simulink model "sampleModel275"  (R2021b)
settings: Solver=VariableStepAuto  StartTime=0.0  StopTime=10.0  RelTol=1e-3
undefined symbols (not defined in the file or in its folder): DiscIntNeverNeededParam, Newton, Raphson
libraries: simulink x15, slpidlib x3
settings Model: Creator=user  LastModifiedBy=user

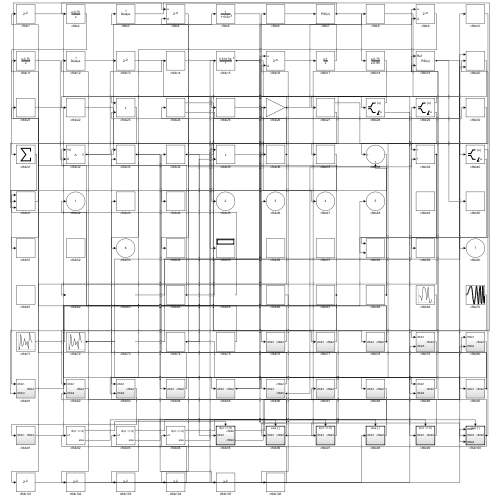
[thumbnail: Simulink's stored preview of the top-level diagram]
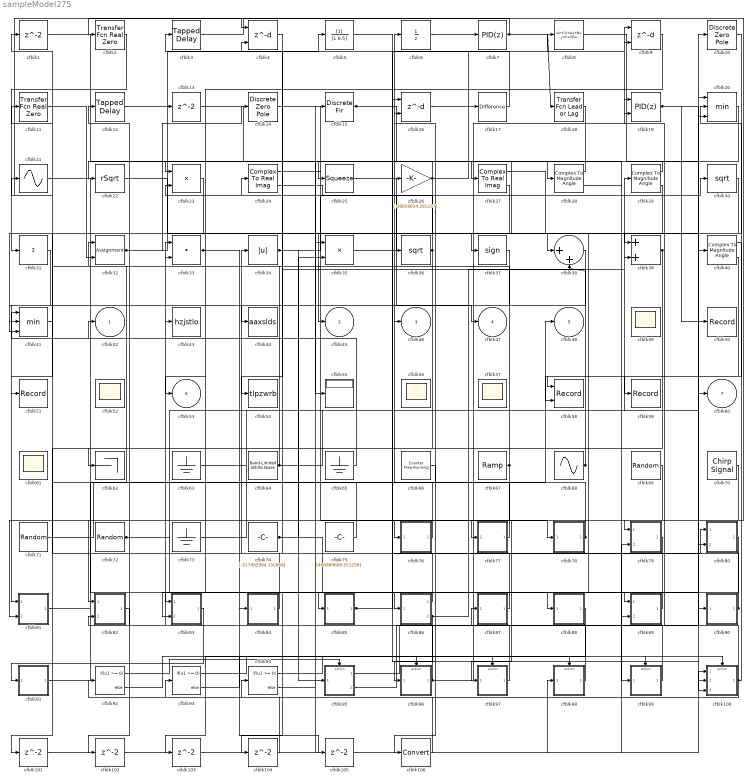
== system sampleModel275 ==
  cfblk{1,13,101..105} (7 alike) : Delay  SampleTime=1
  cfblk10 : DiscreteZeroPole  Poles=[0 0.5]  Gain=1
  cfblk100 : Subsystem  TreatAsAtomicUnit=on
  cfblk106 : DataTypeConversion
  cfblk11 : simulink/Discrete/Transfer Fcn Real Zero  ZeroZ=0.75  ICPrevInput=0.0  DoSatur=off
      settings: SourceProductBaseCode=SL
  cfblk12 : simulink/Discrete/Tapped Delay  vinit=0.0  samptime=-1  NumDelays=1  DelayOrder=Oldest  includeCurrent=off
  cfblk14 : DiscreteZeroPole  Poles=[0 0.5]  Gain=1
  cfblk15 : DiscreteFir  SampleTime=1
  cfblk16 : Delay  DelayLengthSource=Input port  SampleTime=1
      settings: InputPortMap=u0,p1
  cfblk17 : simulink/Discrete/Difference  ICPrevInput=0.0  OutMin=[]  OutMax=[]  OutDataTypeStr=Inherit: Inherit via back propagation  OutDataType=fixdt(1, 16)  OutScaling=2^-10  DoSatur=off
  cfblk18 : simulink/Discrete/Transfer Fcn Lead or Lag  PoleZ=0.95  ZeroZ=0.75  ICPrevOutput=0.0  ICPrevInput=0.0  DoSatur=off
      settings: SourceProductBaseCode=SL
  cfblk19 : slpidlib/PID Controller (2DOF)  Controller=PID  Form=Parallel  TimeDomain=Discrete-time  UseExternalTs=off  SampleTime=1  IntegratorMethod=Forward Euler  FilterMethod=Forward Euler  ControllerParametersSource=internal  P=1  I=1  D=0  UseFilter=on  N=100  b=1  c=1  TunerSelectOption=Transfer Function Based (PID Tuner App)  InitialConditionSource=internal  InitialConditionForIntegrator=0  InitialConditionForFilter=0  DifferentiatorICPrevScaledInput=0  ExternalReset=none  TrackingMode=off  Kt=1  LimitOutput=off  SatLimitsSource=internal  UpperSaturationLimit=inf  LowerSaturationLimit=-inf  LinearizeAsGain=off  AntiWindupMode=none  Kb=1  POutMin=[]  POutMax=[]  IOutMin=[]  IOutMax=[]  DOutMin=[]  DOutMax=[]  NOutMin=[]  NOutMax=[]  bOutMin=[]  bOutMax=[]  cOutMin=[]  cOutMax=[]  SumOutMin=[]  SumOutMax=[]  SaturationOutMin=[]  SaturationOutMax=[]  PParamMin=[]  PParamMax=[]  IParamMin=[]  IParamMax=[]  DParamMin=[]  DParamMax=[]  NParamMin=[]  NParamMax=[]  bParamMin=[]  bParamMax=[]  cParamMin=[]  cParamMax=[]  KbParamMin=[]  KbParamMax=[]  KtParamMin=[]  KtParamMax=[]  KbOutMin=[]  KbOutMax=[]  KtOutMin=[]  KtOutMax=[]  IntegratorOutMin=[]  IntegratorOutMax=[]  FilterOutMin=[]  FilterOutMax=[]  SumI1OutMin=[]  SumI1OutMax=[]  SumI2OutMin=[]  SumI2OutMax=[]  SumI3OutMin=[]  SumI3OutMax=[]  SumI4OutMin=[]  SumI4OutMax=[]  SumDOutMin=[]  SumDOutMax=[]  Sum1OutMin=[]  Sum1OutMax=[]  Sum2OutMin=[]  Sum2OutMax=[]  Sum3OutMin=[]  Sum3OutMax=[]  DifferentiatorOutMin=[]  DifferentiatorOutMax=[]  FilterDiffOutCoefMin=[]  FilterDiffOutCoefMax=[]  ReciprocalOutMin=[]  ReciprocalOutMax=[]  SumDenOutMin=[]  SumDenOutMax=[]  SumNumOutMin=[]  SumNumOutMax=[]  DivideOutMin=[]  DivideOutMax=[]  UdiffTsProdOutMin=[]  UdiffTsProdOutMax=[]  NTsProdOutMin=[]  NTsProdOutMax=[]  UintegralTsProdOutMin=[]  UintegralTsProdOutMax=[]  UngainTsProdOutMin=[]  UngainTsProdOutMax=[]  IntegratorContinuousStateAttributes=''  IntegratorStateMustResolveToSignalObject=off  IntegratorRTWStateStorageClass=Auto  FilterContinuousStateAttributes=''  FilterStateMustResolveToSignalObject=off  FilterRTWStateStorageClass=Auto  ParallelPVariant=InternalParameters  IdealPVariant=Disabled  IVariant=InternalParameters  DVariant=InternalParameters  bVariant=InternalParameters  cVariant=InternalParameters  IntegratorVariant=Discrete  SatVariant=Disabled  AWVariant=Passthrough  PCopyVariant=Disabled  TRVariant=Disabled  FdbkBlocksVariant=Forward  IdealPFdbkVariant=Disabled  SatFdbkVariant=Disabled  DerivativeFilterVariant=ForwardEulerFilter  NVariant=InternalParameters  NCopyVariant=Disabled  FilterICVariant=InternalICsFilter  IntegratorICVariant=InternalICs  ExternalResetVariant=Disabled  TRSumVariant=Passthrough  SumFdbkVariant=Disabled  SumVariant=Sum_PID  TsampFilterVariant=InternalTs  TsampNgainVariant=Passthrough  TsampIntegralVariant=Passthrough  ExternalSaturationOutDataTypeStr=Inherit: Same as second input
      settings: SourceProductBaseCode=SL
  cfblk2 : simulink/Discrete/Transfer Fcn Real Zero  ZeroZ=0.75  ICPrevInput=0.0  DoSatur=off
      settings: SourceProductBaseCode=SL
  cfblk20 : MinMax  Inputs=3
  cfblk21 : Sin  TimeSource=Use external signal  SampleTime=0
  cfblk22 : Sqrt  Operator=rSqrt  AlgorithmType=Newton-Raphson  SaturateOnIntegerOverflow=on
  cfblk23 : Product
  cfblk24 : ComplexToRealImag
  cfblk25 : Squeeze
  cfblk26 : Gain  Gain=[-28658814.291237]
  cfblk27 : ComplexToRealImag
  cfblk28 : ComplexToMagnitudeAngle
  cfblk29 : ComplexToMagnitudeAngle
  cfblk3 : simulink/Discrete/Tapped Delay  vinit=0.0  samptime=-1  NumDelays=1  DelayOrder=Oldest  includeCurrent=off
  cfblk30 : Sqrt  SaturateOnIntegerOverflow=on
  cfblk31 : Sum  Inputs=+
  cfblk32 : Assignment  DiagnosticForDimensions=Warning  IndexOptions=Index vector (dialog)  Indices=1  OutputSizes=1
  cfblk33 : DotProduct  InputSameDT=on  OutDataTypeStr=Inherit: Inherit via internal rule
  cfblk34 : Abs
  cfblk35 : Product  Inputs=**
  cfblk36 : Sqrt  SaturateOnIntegerOverflow=on
  cfblk37 : Signum
  cfblk38 : Sum  Inputs=|++
  cfblk39 : Sum
  cfblk4 : Delay  DelayLengthSource=Input port  SampleTime=1
      settings: InputPortMap=u0,p1
  cfblk40 : ComplexToMagnitudeAngle
  cfblk41 : MinMax  Inputs=3
  cfblk43 : ToWorkspace  VariableName=hzjstlo  SaveFormat=Timeseries  SampleTime=-1
  cfblk44 : ToWorkspace  VariableName=aaxslds  SaveFormat=Timeseries  SampleTime=-1
  cfblk{49,52,56..57,61} (5 alike) : Scope
      settings: Floating=on
  cfblk5 : DiscreteFilter  SampleTime=1
  cfblk50 : Record  FileSettingsInternal="{\"entries\":[{\"content\":{\"excelSettings\":{\"content\":{},\"type\":\"Streamout.ExcelSettings\"}},\"type\":\"Streamout.FileSettingStorage\",\"uuid\":\"b6eb8a9c-eb1a-4261-9b81-98630c569aa1\"}],\"packageUris\":[\"http://schema.mathworks.com/mf0/streamout_blocks/R2020a\"],\"version\":\"1.0\"}"  SignalsInternal="{\"entries\":[{\"content\":{\"signals\":[{\"content\":{\"blockPath\":[\"sampleModel275/cfblk50\"],\"channel\":[],\"dimensions\":[1],\"domain\":\"sampleModel275/cfblk50\",\"lineColor\":\"#fe330a\",\"plots\":[1],\"port\":1,\"sid\":[\"\"],\"signalID\":11495,\"signalName\":\"cfblk19\"},\"type\":\"RecordBlkView.Signal\",\"uuid\":\"71f57f67-cb61-4adf-8332-56198fc03cd2\"}]},\"type\":\"RecordBlkView.InputSignals\",\"uuid\":\"8c8ca269-4e9b-46e2-88c4-c1c2e234a8b1\"}],\"packageUris\":[\"http://schema.mathworks.com/mf0/streamout_blocks/R2020a\"],\"version\":\"1.0\"}"  VisualizationBindings="{\"sparklinesplugin\":{\"info\":[{\"bindingParametersList\":[],\"subplotID\":1}]}}"
  cfblk51 : Record  FileSettingsInternal="{\"entries\":[{\"content\":{\"excelSettings\":{\"content\":{},\"type\":\"Streamout.ExcelSettings\"}},\"type\":\"Streamout.FileSettingStorage\",\"uuid\":\"b407e88e-82d7-4c58-97ca-e59b3c794d53\"}],\"packageUris\":[\"http://schema.mathworks.com/mf0/streamout_blocks/R2020a\"],\"version\":\"1.0\"}"  SignalsInternal="{\"entries\":[{\"content\":{\"signals\":[{\"content\":{\"blockPath\":[\"sampleModel275/cfblk51\"],\"channel\":[],\"dimensions\":[1],\"domain\":\"sampleModel275/cfblk51\",\"lineColor\":\"#22b573\",\"plots\":[1],\"port\":1,\"sid\":[\"\"],\"signalID\":11499,\"signalName\":\"cfblk23\"},\"type\":\"RecordBlkView.Signal\",\"uuid\":\"ec15170a-8382-47db-b36d-1ce41cc8f111\"}]},\"type\":\"RecordBlkView.InputSignals\",\"uuid\":\"f86542a5-57eb-4307-8b55-610ba7e4df7d\"}],\"packageUris\":[\"http://schema.mathworks.com/mf0/streamout_blocks/R2020a\"],\"version\":\"1.0\"}"  VisualizationBindings="{\"sparklinesplugin\":{\"info\":[{\"bindingParametersList\":[],\"subplotID\":1}]}}"
  cfblk54 : ToWorkspace  VariableName=tlpzwrb  SaveFormat=Timeseries  SampleTime=-1
  cfblk55 : Display
  cfblk58 : Record  FileSettingsInternal="{\"entries\":[{\"content\":{\"excelSettings\":{\"content\":{},\"type\":\"Streamout.ExcelSettings\"}},\"type\":\"Streamout.FileSettingStorage\",\"uuid\":\"6438ada9-0782-4b46-9d9c-291e916b62cd\"}],\"packageUris\":[\"http://schema.mathworks.com/mf0/streamout_blocks/R2020a\"],\"version\":\"1.0\"}"  Layout=[1 1]  SignalsInternal="{\"entries\":[{\"content\":{\"signals\":[{\"content\":{\"blockPath\":[\"sampleModel275/cfblk58\"],\"channel\":[],\"dimensions\":[1],\"domain\":\"sampleModel275/cfblk58\",\"lineColor\":\"#a2142f\",\"plots\":[1],\"port\":1,\"sid\":[\"\"],\"signalID\":11503,\"signalName\":\"cfblk40:1\"},\"type\":\"RecordBlkView.Signal\",\"uuid\":\"d4910d3c-664b-4734-92f5-20726efe3d51\"},{\"content\":{\"blockPath\":[\"sampleModel275/cfblk58\"],\"channel\":[],\"dimensions\":[1],\"domain\":\"sampleModel275/cfblk58\",\"lineColor\":\"#139fff\",\"plots\":[1],\"port\":2,\"sid\":[\"\"],\"signalID\":11507,\"signalName\":\"cfblk39\"},\"type\":\"RecordBlkView.Signal\",\"uuid\":\"d5fbbb1f-5277-447b-a33f-a90c886777ef\"}]},\"type\":\"RecordBlkView.InputSignals\",\"uuid\":\"5aa0f4f9-8f77-40f4-b90e-7cbebfc535ff\"}],\"packageUris\":[\"http://schema.mathworks.com/mf0/streamout_blocks/R2020a\"],\"version\":\"1.0\"}"  VisualizationBindings="{\"xyplotplugin\":{\"info\":[{\"series\":[{\"bindingParametersList\":[{\"parameter\":\"X-Axis\",\"signalID\":11503,\"signalName\":\"cfblk40:1\"},{\"parameter\":\"Y-Axis\",\"signalID\":11507,\"signalName\":\"cfblk39\"}],\"seriesID\":64902}],\"subplotID\":1}]}}"  CompatibilityTag=XY
  cfblk59 : Record  FileSettingsInternal="{\"entries\":[{\"content\":{\"excelSettings\":{\"content\":{},\"type\":\"Streamout.ExcelSettings\"}},\"type\":\"Streamout.FileSettingStorage\",\"uuid\":\"0cc106a6-c31f-4d23-977d-6d8b87a6092b\"}],\"packageUris\":[\"http://schema.mathworks.com/mf0/streamout_blocks/R2020a\"],\"version\":\"1.0\"}"  SignalsInternal="{\"entries\":[{\"content\":{\"signals\":[{\"content\":{\"blockPath\":[\"sampleModel275/cfblk59\"],\"channel\":[],\"dimensions\":[1],\"domain\":\"sampleModel275/cfblk59\",\"lineColor\":\"#edb120\",\"plots\":[1],\"port\":1,\"sid\":[\"\"],\"signalID\":11511,\"signalName\":\"cfblk40:2\"},\"type\":\"RecordBlkView.Signal\",\"uuid\":\"fdcc7cc7-3bfd-4a9a-aeaa-3b1704c8eba9\"}]},\"type\":\"RecordBlkView.InputSignals\",\"uuid\":\"85a8b503-552f-41f1-b276-6a567ca8898e\"}],\"packageUris\":[\"http://schema.mathworks.com/mf0/streamout_blocks/R2020a\"],\"version\":\"1.0\"}"  VisualizationBindings="{\"sparklinesplugin\":{\"info\":[{\"bindingParametersList\":[],\"subplotID\":1}]}}"
  cfblk6 : UnitDelay  HasFrameUpgradeWarning=on
  cfblk62 : Terminator
  cfblk63 : Ground
  cfblk64 : simulink/Sources/Band-Limited White Noise  Cov=[1822602826.106394]  Ts=0.1  seed=[609401567.000000]
  cfblk65 : Ground
  cfblk66 : simulink/Sources/Counter Free-Running  NumBits=[2.000000]  tsamp=-1
  cfblk67 : simulink/Sources/Ramp  slope=[-6244.976226]  start=[33.233688]  InitialOutput=[-507448.704039]
  cfblk68 : Sin  Amplitude=[-991310042.468495]  Bias=[911881758.142677]  SampleTime=0
  cfblk69 : RandomNumber  Mean=[-38034.714186]  Variance=[20282.555075]  Seed=[711987577.000000]  SampleTime=0.1
  cfblk7 : slpidlib/PID Controller  Controller=PID  Form=Parallel  TimeDomain=Discrete-time  UseExternalTs=off  SampleTime=1  IntegratorMethod=Forward Euler  FilterMethod=Forward Euler  ControllerParametersSource=internal  P=1  I=1  D=0  UseFilter=on  N=100  TunerSelectOption=Transfer Function Based (PID Tuner App)  InitialConditionSource=internal  InitialConditionForIntegrator=0  InitialConditionForFilter=0  DifferentiatorICPrevScaledInput=0  ExternalReset=none  TrackingMode=off  Kt=1  LimitOutput=off  SatLimitsSource=internal  UpperSaturationLimit=inf  LowerSaturationLimit=-inf  LinearizeAsGain=off  AntiWindupMode=none  Kb=1  POutMin=[]  POutMax=[]  IOutMin=[]  IOutMax=[]  DOutMin=[]  DOutMax=[]  NOutMin=[]  NOutMax=[]  SumOutMin=[]  SumOutMax=[]  SaturationOutMin=[]  SaturationOutMax=[]  PParamMin=[]  PParamMax=[]  IParamMin=[]  IParamMax=[]  DParamMin=[]  DParamMax=[]  NParamMin=[]  NParamMax=[]  KbParamMin=[]  KbParamMax=[]  KtParamMin=[]  KtParamMax=[]  KbOutMin=[]  KbOutMax=[]  KtOutMin=[]  KtOutMax=[]  IntegratorOutMin=[]  IntegratorOutMax=[]  FilterOutMin=[]  FilterOutMax=[]  SumI1OutMin=[]  SumI1OutMax=[]  SumI2OutMin=[]  SumI2OutMax=[]  SumI3OutMin=[]  SumI3OutMax=[]  SumI4OutMin=[]  SumI4OutMax=[]  SumDOutMin=[]  SumDOutMax=[]  DifferentiatorOutMin=[]  DifferentiatorOutMax=[]  FilterDiffOutCoefMin=[]  FilterDiffOutCoefMax=[]  ReciprocalOutMin=[]  ReciprocalOutMax=[]  SumDenOutMin=[]  SumDenOutMax=[]  SumNumOutMin=[]  SumNumOutMax=[]  DivideOutMin=[]  DivideOutMax=[]  UdiffTsProdOutMin=[]  UdiffTsProdOutMax=[]  NTsProdOutMin=[]  NTsProdOutMax=[]  UintegralTsProdOutMin=[]  UintegralTsProdOutMax=[]  UngainTsProdOutMin=[]  UngainTsProdOutMax=[]  IntegratorContinuousStateAttributes=''  IntegratorStateMustResolveToSignalObject=off  IntegratorRTWStateStorageClass=Auto  FilterContinuousStateAttributes=''  FilterStateMustResolveToSignalObject=off  FilterRTWStateStorageClass=Auto  ParallelPVariant=InternalParameters  IdealPVariant=Disabled  IVariant=InternalParameters  DVariant=InternalParameters  IntegratorVariant=Discrete  SatVariant=Disabled  AWVariant=Passthrough  PCopyVariant=Disabled  TRVariant=Disabled  FdbkBlocksVariant=Forward  IdealPFdbkVariant=Disabled  SatFdbkVariant=Disabled  DerivativeFilterVariant=ForwardEulerFilter  NVariant=InternalParameters  NCopyVariant=Disabled  FilterICVariant=InternalICsFilter  IntegratorICVariant=InternalICs  ExternalResetVariant=Disabled  TRSumVariant=Passthrough  SumFdbkVariant=Disabled  SumVariant=Sum_PID  TsampFilterVariant=InternalTs  TsampNgainVariant=Passthrough  TsampIntegralVariant=Passthrough  ExternalSaturationOutDataTypeStr=Inherit: Same as second input
  cfblk70 : simulink/Sources/Chirp Signal  f1=[-497496428.255799]  T=[-926255871.400772]  f2=[-805731715.239342]
  cfblk71 : UniformRandomNumber  Minimum=[-1039848184.369478]  Maximum=[7342485115.905728]  Seed=[43463213.000000]  SampleTime=0.1
  cfblk72 : UniformRandomNumber  Minimum=[-2028484056.447849]  Maximum=[4927057979.813775]  Seed=[54197265.000000]  SampleTime=0.1
  cfblk73 : Ground
  cfblk74 : Constant  Value=[-527492994.150068]  SampleTime=1
  cfblk75 : Constant  Value=[406889608.551256]  SampleTime=1
  cfblk76 : Subsystem
  cfblk77 : Subsystem
  cfblk78 : Subsystem
  cfblk79 : Subsystem
  cfblk8 : DiscreteStateSpace
  cfblk80 : Subsystem
  cfblk81 : Subsystem
  cfblk82 : Subsystem
  cfblk83 : Subsystem
  cfblk84 : Subsystem
  cfblk85 : Subsystem
  cfblk86 : Subsystem
  cfblk87 : Subsystem
  cfblk88 : Subsystem
  cfblk89 : Subsystem
  cfblk9 : Delay  DelayLengthSource=Input port  SampleTime=1
      settings: InputPortMap=u0,p1
  cfblk90 : Subsystem
  cfblk91 : Subsystem
  cfblk92 : If  IfExpression=u1 >= 0  SampleTime=1
  cfblk93 : If  IfExpression=u1 >= 0  SampleTime=1
  cfblk94 : If  IfExpression=u1 >= 0  SampleTime=1
  cfblk95 : Subsystem  TreatAsAtomicUnit=on
  cfblk96 : Subsystem  TreatAsAtomicUnit=on
  cfblk97 : Subsystem  TreatAsAtomicUnit=on
  cfblk98 : Subsystem  TreatAsAtomicUnit=on
  cfblk99 : Subsystem  TreatAsAtomicUnit=on
  cfblk42 : Outport
  cfblk45 : Outport  Port=2
  cfblk46 : Outport  Port=3
  cfblk47 : Outport  Port=4
  cfblk48 : Outport  Port=5
  cfblk53 : Outport  Port=6
  cfblk60 : Outport  Port=7
  wires:
  cfblk17/1 -> cfblk3/1
  cfblk40/1 -> cfblk58/1
  cfblk21/1 -> cfblk85/1(cfblk1)
  cfblk96/1(cfblk2) -> cfblk9/1, cfblk82/2(cfblk4)
  cfblk71/1 -> cfblk48/1
  cfblk89/1(cfblk2) -> cfblk86/1(cfblk1)
  cfblk34/1 -> cfblk30/1, cfblk95/1(cfblk1)
  cfblk84/1(cfblk2) -> cfblk34/1
  cfblk3/1 -> cfblk79/1(cfblk1)
  cfblk24/1 -> cfblk76/1(cfblk1)
  cfblk10/1 -> cfblk38/1
  cfblk18/1 -> cfblk27/1
  cfblk14/1 -> cfblk77/1(cfblk1)
  cfblk32/1 -> cfblk5/1, cfblk14/1
  cfblk19/1 -> cfblk40/1, cfblk50/1
  cfblk73/1 -> cfblk6/1
  cfblk63/1 -> cfblk29/1
  cfblk20/1 -> cfblk37/1
  cfblk25/1 -> cfblk47/1
  cfblk24/2 -> cfblk26/1
  cfblk31/1 -> cfblk81/1(cfblk1)
  cfblk4/1 -> cfblk54/1
  cfblk97/1(cfblk2) -> cfblk33/1
  cfblk36/1 -> cfblk91/1(cfblk1), cfblk23/2
  cfblk37/1 -> cfblk44/1
  cfblk30/1 -> cfblk88/1(cfblk1)
  cfblk41/1 -> cfblk4/1
  cfblk90/1(cfblk2) -> cfblk4/2, cfblk19/2
  cfblk9/1 -> cfblk83/1(cfblk1)
  cfblk2/1 -> cfblk31/1
  cfblk65/1 -> cfblk41/1
  cfblk1/1 -> cfblk28/1
  cfblk39/1 -> cfblk62/1, cfblk58/2
  cfblk28/1 -> cfblk22/1
  cfblk33/1 -> cfblk84/1(cfblk1), cfblk105/1
  cfblk76/1(cfblk2) -> cfblk32/1
  cfblk26/1 -> cfblk45/1, cfblk25/1, cfblk9/2
  cfblk98/1(cfblk2) -> cfblk87/1(cfblk1)
  cfblk8/1 -> cfblk60/1
  cfblk67/1 -> cfblk33/2, cfblk82/1(cfblk1)
  cfblk70/1 -> cfblk81/2(cfblk3)
  cfblk87/1(cfblk2) -> cfblk1/1
  cfblk5/1 -> cfblk78/1(cfblk1)
  cfblk69/1 -> cfblk97/1(cfblk1)
  cfblk35/1 -> cfblk10/1
  cfblk22/1 -> cfblk90/1(cfblk1)
  cfblk85/1(cfblk2) -> cfblk80/1(cfblk1), cfblk8/1
  cfblk11/1 -> cfblk32/2
  cfblk23/1 -> cfblk51/1
  cfblk95/1(cfblk2) -> cfblk80/2(cfblk4)
  cfblk99/1(cfblk2) -> cfblk12/1
  cfblk74/1 -> cfblk89/1(cfblk1), cfblk35/2
  cfblk95/2(cfblk4) -> cfblk20/1
  cfblk77/1(cfblk2) -> cfblk46/1
  cfblk40/2 -> cfblk59/1
  cfblk64/1 -> cfblk16/1, cfblk21/1
  cfblk28/2 -> cfblk99/1(cfblk1)
  cfblk38/1 -> cfblk41/2
  cfblk78/1(cfblk2) -> cfblk42/1, cfblk16/2
  cfblk68/1 -> cfblk24/1, cfblk38/2
  cfblk72/1 -> cfblk100/2(cfblk3), cfblk20/3
  cfblk13/1 -> cfblk55/1
  cfblk15/1 -> cfblk89/2(cfblk4), cfblk100/3(cfblk4)
  cfblk6/1 -> cfblk7/1
  cfblk81/1(cfblk2) -> cfblk36/1
  cfblk12/1 -> cfblk13/1
  cfblk91/1(cfblk2) -> cfblk35/1
  cfblk29/1 -> cfblk23/1
  cfblk75/1 -> cfblk11/1
  cfblk27/1 -> cfblk39/1
  cfblk16/1 -> cfblk17/1
  cfblk27/2 -> cfblk41/3
  cfblk79/1(cfblk2) -> cfblk83/2(cfblk4)
  cfblk86/1(cfblk2) -> cfblk43/1
  cfblk29/2 -> cfblk53/1
  cfblk100/1(cfblk2) -> cfblk93/1, cfblk19/1, cfblk20/2
  cfblk86/2(cfblk5) -> cfblk96/1(cfblk1), cfblk39/2
  cfblk7/1 -> cfblk18/1, cfblk2/1
  cfblk92/1 -> cfblk95/Action
  cfblk92/2 -> cfblk96/Action
  cfblk93/1 -> cfblk97/Action
  cfblk93/2 -> cfblk98/Action
  cfblk94/1 -> cfblk99/Action
  cfblk94/2 -> cfblk100/Action
  cfblk83/1(cfblk2) -> cfblk101/1
  cfblk101/1 -> cfblk79/2(cfblk5)
  cfblk82/1(cfblk2) -> cfblk102/1
  cfblk102/1 -> cfblk15/1
  cfblk88/1(cfblk2) -> cfblk103/1
  cfblk103/1 -> cfblk100/1(cfblk1)
  cfblk80/1(cfblk2) -> cfblk104/1
  cfblk104/1 -> cfblk92/1
  cfblk105/1 -> cfblk98/1(cfblk1)
  cfblk66/1 -> cfblk106/1
  cfblk106/1 -> cfblk94/1

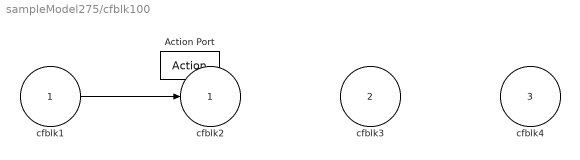
== system sampleModel275/cfblk100 ==
  cfblk1 : Inport
  cfblk3 : Inport  Port=2
  cfblk4 : Inport  Port=3
  Action Port : ActionPort  ActionPortLabel=else
  cfblk2 : Outport
  wires:
  cfblk1/1 -> cfblk2/1

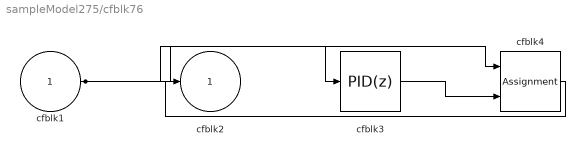
== system sampleModel275/cfblk76 ==
  cfblk1 : Inport
  cfblk3 : slpidlib/PID Controller  Controller=PID  Form=Parallel  TimeDomain=Discrete-time  UseExternalTs=off  SampleTime=1  IntegratorMethod=Forward Euler  FilterMethod=Forward Euler  ControllerParametersSource=internal  P=1  I=1  D=0  UseFilter=on  N=100  TunerSelectOption=Transfer Function Based (PID Tuner App)  InitialConditionSource=internal  InitialConditionForIntegrator=0  InitialConditionForFilter=0  DifferentiatorICPrevScaledInput=0  ExternalReset=none  TrackingMode=off  Kt=1  LimitOutput=off  SatLimitsSource=internal  UpperSaturationLimit=inf  LowerSaturationLimit=-inf  LinearizeAsGain=off  AntiWindupMode=none  Kb=1  POutMin=[]  POutMax=[]  IOutMin=[]  IOutMax=[]  DOutMin=[]  DOutMax=[]  NOutMin=[]  NOutMax=[]  SumOutMin=[]  SumOutMax=[]  SaturationOutMin=[]  SaturationOutMax=[]  PParamMin=[]  PParamMax=[]  IParamMin=[]  IParamMax=[]  DParamMin=[]  DParamMax=[]  NParamMin=[]  NParamMax=[]  KbParamMin=[]  KbParamMax=[]  KtParamMin=[]  KtParamMax=[]  KbOutMin=[]  KbOutMax=[]  KtOutMin=[]  KtOutMax=[]  IntegratorOutMin=[]  IntegratorOutMax=[]  FilterOutMin=[]  FilterOutMax=[]  SumI1OutMin=[]  SumI1OutMax=[]  SumI2OutMin=[]  SumI2OutMax=[]  SumI3OutMin=[]  SumI3OutMax=[]  SumI4OutMin=[]  SumI4OutMax=[]  SumDOutMin=[]  SumDOutMax=[]  DifferentiatorOutMin=[]  DifferentiatorOutMax=[]  FilterDiffOutCoefMin=[]  FilterDiffOutCoefMax=[]  ReciprocalOutMin=[]  ReciprocalOutMax=[]  SumDenOutMin=[]  SumDenOutMax=[]  SumNumOutMin=[]  SumNumOutMax=[]  DivideOutMin=[]  DivideOutMax=[]  UdiffTsProdOutMin=[]  UdiffTsProdOutMax=[]  NTsProdOutMin=[]  NTsProdOutMax=[]  UintegralTsProdOutMin=[]  UintegralTsProdOutMax=[]  UngainTsProdOutMin=[]  UngainTsProdOutMax=[]  IntegratorContinuousStateAttributes=''  IntegratorStateMustResolveToSignalObject=off  IntegratorRTWStateStorageClass=Auto  FilterContinuousStateAttributes=''  FilterStateMustResolveToSignalObject=off  FilterRTWStateStorageClass=Auto  ParallelPVariant=InternalParameters  IdealPVariant=Disabled  IVariant=InternalParameters  DVariant=InternalParameters  IntegratorVariant=Discrete  SatVariant=Disabled  AWVariant=Passthrough  PCopyVariant=Disabled  TRVariant=Disabled  FdbkBlocksVariant=Forward  IdealPFdbkVariant=Disabled  SatFdbkVariant=Disabled  DerivativeFilterVariant=ForwardEulerFilter  NVariant=InternalParameters  NCopyVariant=Disabled  FilterICVariant=InternalICsFilter  IntegratorICVariant=InternalICs  ExternalResetVariant=Disabled  TRSumVariant=Passthrough  SumFdbkVariant=Disabled  SumVariant=Sum_PID  TsampFilterVariant=InternalTs  TsampNgainVariant=Passthrough  TsampIntegralVariant=Passthrough  ExternalSaturationOutDataTypeStr=Inherit: Same as second input
  cfblk4 : Assignment  DiagnosticForDimensions=Warning  IndexOptions=Index vector (dialog)  Indices=1  OutputSizes=1
  cfblk2 : Outport
  wires:
  cfblk1/1 -> cfblk4/1, cfblk3/1
  cfblk4/1 -> cfblk2/1
  cfblk3/1 -> cfblk4/2

== system sampleModel275/cfblk77 ==
  cfblk1 : Inport
  cfblk3 : DiscreteIntegrator  ICPrevOutput=DiscIntNeverNeededParam  ICPrevScaledInput=DiscIntNeverNeededParam
  cfblk2 : Outport
  wires:
  cfblk1/1 -> cfblk2/1, cfblk3/1

== system sampleModel275/cfblk78 ==
  cfblk1 : Inport
  cfblk3 : Polyval  Coefs=[ +2.081618890e-019, -1.441693666e-014, +4.719686976e-010, -8.536869453e-006, +1.621573104e-001, -8.087801117e+001 ]
  cfblk2 : Outport
  wires:
  cfblk3/1 -> cfblk2/1
  cfblk1/1 -> cfblk3/1

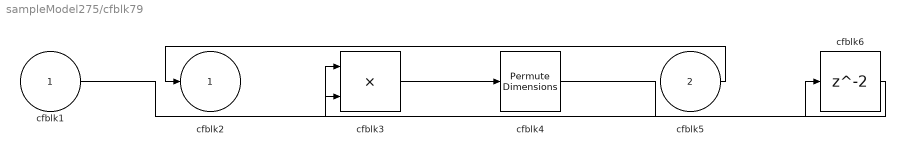
== system sampleModel275/cfblk79 ==
  cfblk1 : Inport
  cfblk5 : Inport  Port=2
  cfblk3 : Product
  cfblk4 : PermuteDimensions
  cfblk6 : Delay  SampleTime=1
  cfblk2 : Outport
  wires:
  cfblk5/1 -> cfblk2/1
  cfblk1/1 -> cfblk3/1
  cfblk3/1 -> cfblk4/1
  cfblk4/1 -> cfblk6/1
  cfblk6/1 -> cfblk3/2

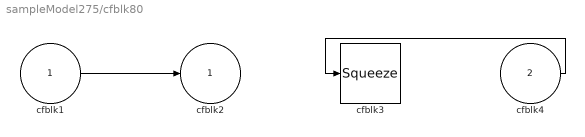
== system sampleModel275/cfblk80 ==
  cfblk1 : Inport
  cfblk4 : Inport  Port=2
  cfblk3 : Squeeze
  cfblk2 : Outport
  wires:
  cfblk4/1 -> cfblk3/1
  cfblk1/1 -> cfblk2/1

== system sampleModel275/cfblk81 ==
  cfblk1 : Inport
  cfblk3 : Inport  Port=2
  cfblk2 : Outport
  wires:
  cfblk1/1 -> cfblk2/1

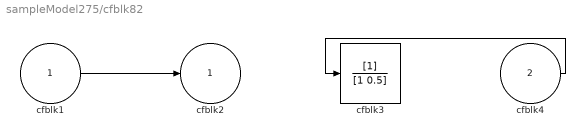
== system sampleModel275/cfblk82 ==
  cfblk1 : Inport
  cfblk4 : Inport  Port=2
  cfblk3 : DiscreteFilter  SampleTime=1
  cfblk2 : Outport
  wires:
  cfblk4/1 -> cfblk3/1
  cfblk1/1 -> cfblk2/1

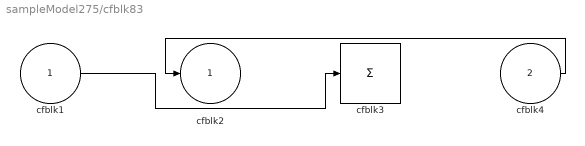
== system sampleModel275/cfblk83 ==
  cfblk1 : Inport
  cfblk4 : Inport  Port=2
  cfblk3 : Sum  Inputs=+
  cfblk2 : Outport
  wires:
  cfblk4/1 -> cfblk2/1
  cfblk1/1 -> cfblk3/1

== system sampleModel275/cfblk84 ==
  cfblk1 : Inport
  cfblk3 : simulink/Math Operations/MinMax Running Resettable  Function=min  vinit=0.0
  cfblk2 : Outport
  wires:
  cfblk1/1 -> cfblk3/1, cfblk3/2
  cfblk3/1 -> cfblk2/1

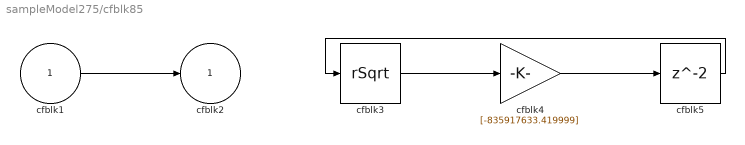
== system sampleModel275/cfblk85 ==
  cfblk1 : Inport
  cfblk3 : Sqrt  Operator=rSqrt  AlgorithmType=Newton-Raphson  SaturateOnIntegerOverflow=on
  cfblk4 : Gain  Gain=[-835917633.419999]
  cfblk5 : Delay  SampleTime=1
  cfblk2 : Outport
  wires:
  cfblk3/1 -> cfblk4/1
  cfblk1/1 -> cfblk2/1
  cfblk4/1 -> cfblk5/1
  cfblk5/1 -> cfblk3/1

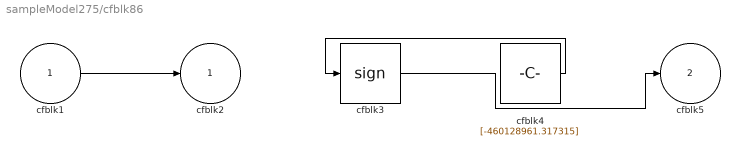
== system sampleModel275/cfblk86 ==
  cfblk1 : Inport
  cfblk3 : Signum
  cfblk4 : Constant  Value=[-460128961.317315]  SampleTime=1
  cfblk2 : Outport
  cfblk5 : Outport  Port=2
  wires:
  cfblk4/1 -> cfblk3/1
  cfblk3/1 -> cfblk5/1
  cfblk1/1 -> cfblk2/1

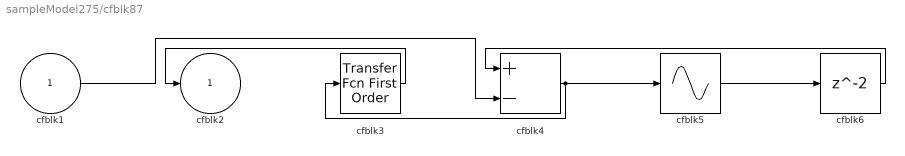
== system sampleModel275/cfblk87 ==
  cfblk1 : Inport
  cfblk3 : simulink/Discrete/Transfer Fcn First Order  PoleZ=0.95  ICPrevOutput=0.0  DoSatur=off
  cfblk4 : Sum  Inputs=+-
  cfblk5 : Sin  TimeSource=Use external signal  SampleTime=0
  cfblk6 : Delay  SampleTime=1
  cfblk2 : Outport
  wires:
  cfblk3/1 -> cfblk2/1
  cfblk4/1 -> cfblk3/1, cfblk5/1
  cfblk1/1 -> cfblk4/2
  cfblk5/1 -> cfblk6/1
  cfblk6/1 -> cfblk4/1

== system sampleModel275/cfblk88 ==
  cfblk1 : Inport
  cfblk3 : ComplexToRealImag
  cfblk2 : Outport
  wires:
  cfblk1/1 -> cfblk3/1
  cfblk3/1 -> cfblk2/1

== system sampleModel275/cfblk89 ==
  cfblk1 : Inport
  cfblk4 : Inport  Port=2
  cfblk3 : Product
  cfblk2 : Outport
  wires:
  cfblk3/1 -> cfblk2/1
  cfblk1/1 -> cfblk3/1
  cfblk4/1 -> cfblk3/2

== system sampleModel275/cfblk90 ==
  cfblk1 : Inport
  cfblk3 : Sin  TimeSource=Use external signal  SampleTime=0
  cfblk2 : Outport
  wires:
  cfblk3/1 -> cfblk2/1
  cfblk1/1 -> cfblk3/1

== system sampleModel275/cfblk91 ==
  cfblk1 : Inport
  cfblk3 : simulink/Discrete/Tapped Delay  vinit=0.0  samptime=-1  NumDelays=1  DelayOrder=Oldest  includeCurrent=off
  cfblk4 : Constant  Value=[-924142526.306234]  SampleTime=1
  cfblk2 : Outport
  wires:
  cfblk4/1 -> cfblk3/1
  cfblk1/1 -> cfblk2/1

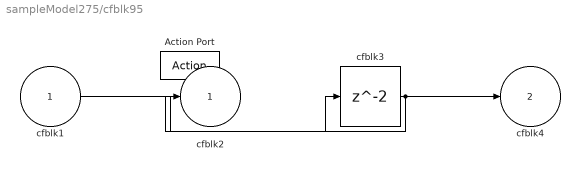
== system sampleModel275/cfblk95 ==
  cfblk1 : Inport
  Action Port : ActionPort  ActionPortLabel=if(u1 >= 0)
  cfblk3 : Delay
  cfblk2 : Outport
  cfblk4 : Outport  Port=2
  wires:
  cfblk3/1 -> cfblk4/1, cfblk2/1
  cfblk1/1 -> cfblk3/1

== system sampleModel275/cfblk96 ==
  cfblk1 : Inport
  Action Port : ActionPort  ActionPortLabel=else
  cfblk3 : Constant  Value=[-629349395.629615]  SampleTime=1
  cfblk2 : Outport
  wires:
  cfblk1/1 -> cfblk2/1

== system sampleModel275/cfblk97 ==
  cfblk1 : Inport
  Action Port : ActionPort  ActionPortLabel=if(u1 >= 0)
  cfblk3 : Rounding
  cfblk2 : Outport
  wires:
  cfblk3/1 -> cfblk2/1
  cfblk1/1 -> cfblk3/1

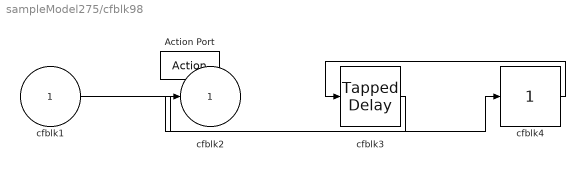
== system sampleModel275/cfblk98 ==
  cfblk1 : Inport
  Action Port : ActionPort  ActionPortLabel=else
  cfblk3 : simulink/Discrete/Tapped Delay  vinit=0.0  samptime=-1  NumDelays=1  DelayOrder=Oldest  includeCurrent=off
  cfblk4 : simulink/Math Operations/Slider Gain  gain=1  low=0  high=2
  cfblk2 : Outport
  wires:
  cfblk4/1 -> cfblk3/1
  cfblk1/1 -> cfblk4/1
  cfblk3/1 -> cfblk2/1

== system sampleModel275/cfblk99 ==
  cfblk1 : Inport
  Action Port : ActionPort  ActionPortLabel=if(u1 >= 0)
  cfblk3 : Constant  Value=[-740095778.448201]  SampleTime=1
  cfblk2 : Outport
  wires:
  cfblk3/1 -> cfblk2/1
